simulink model "ISReferenceApplication"  (R2024b)
settings: Solver=ode5  StartTime=0.0  StopTime=20  FixedStep=1e-3  RelTol=2e-1
model workspace (MAT data in the model file):
  Downshift_Speeds = [9.5625 12.9375 16.3125 19.6875 23.0625 26.4375 29.8125 33.1875 36.5625 39.9375 43.3125 46.6875 ... (28 elements, 4x7)]
  EngRevLim = 7000
  Pedal_Positions = [0.1 0.4 0.5 0.9]
  Upshift_Speeds = [12.9375 16.3125 19.6875 33 26.4375 29.8125 33.1875 52.5 39.9375 43.3125 46.6875 77.25 ... (28 elements, 4x7)]
  VEH : object (value not decoded)
  rayDirections = [0 0 0 0 0 0 0 0 0 0 0 0 ... (363 elements, 121x3)]
  rayLengths = [20 20 20 20 20 20 20 20 20 20 20 20 ... (121 elements, 121x1)]
  rayOrigins = [0.5 0.4 0.3 0.2 0.1 0 -0.1 -0.2 -0.3 -0.4 -0.5 0.5 ... (363 elements, 121x3)]
  temp : object (value not decoded)
symbols that are objects in the model workspace (value not decoded): temp, VEH
undefined symbols (not defined in the file or in its folder): DiscIntNeverNeededParam, Sim3dSensor
libraries: simulink x28, autolibutils x14, VDriveToolbox x10, vehdynlibviscommon x4, sim3dgroundtruthsensorlib x4, slpidlib x3, autolibtranscontrolscommon x2, autolibshared x2, vehdynlibdriver x2, sharedtransform x2, vehdynlibsens x2, vehdynlibscenariocommon x2
(part 7 of 7)

== matlab function ISReferenceApplication/Visualization1/MATLAB Function ==
  data: pos input; agl input; vel input; wheel_agl input; T_ref input; track_w input; a input; b input; diameter input
function XYplot(pos,agl,vel,wheel_agl,T_ref,track_w,a,b,diameter)
persistent fig_xy ref_p
if isempty(fig_xy)
    fig_xy = figure();
    ref_p = plot(-T_ref(:,2),T_ref(:,1),'Color','red','LineWidth',1.5,'DisplayName','Ref. Path'); hold on;
end
body_yaw = agl(3);
body_x = pos(1);
body_y = pos(2);
wfl_x = body_x+a;
wfl_y = body_y-track_w/2;
wfr_x = body_x+a;
wfr_y = body_y+track_w/2;
wrl_x = body_x-b;
wrl_y = body_y-track_w/2;
wrr_x = body_x-b;
wrr_y = body_y+track_w/2;

R_whl = [cos(-wheel_agl(1)) -sin(-wheel_agl(1)) ;sin(-wheel_agl(1)) cos(-wheel_agl(1))];
R_bdy = [cos(-body_yaw) -sin(-body_yaw) ;sin(-body_yaw) cos(-body_yaw)];

wfl_rec_x = [wfl_y-0.1 wfl_y+0.1 wfl_y+0.1 wfl_y-0.1];
wfl_rec_y = [wfl_x-diameter/2 wfl_x-diameter/2 wfl_x+diameter/2 wfl_x+diameter/2];
wfr_rec_x = [wfr_y-0.1 wfr_y+0.1 wfr_y+0.1 wfr_y-0.1];
wfr_rec_y = [wfr_x-diameter/2 wfr_x-diameter/2 wfr_x+diameter/2 wfr_x+diameter/2];
wrl_rec_x = [wrl_y-0.1 wrl_y+0.1 wrl_y+0.1 wrl_y-0.1];
wrl_rec_y = [wrl_x-diameter/2 wrl_x-diameter/2 wrl_x+diameter/2 wrl_x+diameter/2];
wrr_rec_x = [wrr_y-0.1 wrr_y+0.1 wrr_y+0.1 wrr_y-0.1];
wrr_rec_y = [wrr_x-diameter/2 wrr_x-diameter/2 wrr_x+diameter/2 wrr_x+diameter/2];
bdy_rec_x = [body_y-1.731/2 body_y+1.731/2 body_y+1.731/2 body_y-1.731/2];
bdy_rec_y = [body_x-4.769/2 body_x-4.769/2 body_x+4.769/2 body_x+4.769/2];

wfl_rec = [wfl_rec_x;wfl_rec_y];
wfr_rec = [wfr_rec_x;wfr_rec_y];
wrl_rec = [wrl_rec_x;wrl_rec_y];
wrr_rec = [wrr_rec_x;wrr_rec_y];
bdy_rec = [bdy_rec_x;bdy_rec_y];

for i=1:4
    wfl_rec(:,i) = R_whl*(wfl_rec(:,i)-[wfl_y;wfl_x]) + [wfl_y;wfl_x];
    wfr_rec(:,i) = R_whl*(wfr_rec(:,i)-[wfr_y;wfr_x]) + [wfr_y;wfr_x];

    wfl_rec(:,i) = R_bdy*(wfl_rec(:,i)-[body_y;body_x]) + [body_y;body_x];
    wfr_rec(:,i) = R_bdy*(wfr_rec(:,i)-[body_y;body_x]) + [body_y;body_x];
    wrl_rec(:,i) = R_bdy*(wrl_rec(:,i)-[body_y;body_x]) + [body_y;body_x];
    wrr_rec(:,i) = R_bdy*(wrr_rec(:,i)-[body_y;body_x]) + [body_y;body_x];
    bdy_rec(:,i) = R_bdy*(bdy_rec(:,i)-[body_y;body_x]) + [body_y;body_x];
end

hold on;
bdy_sc = scatter(body_y,body_x,10,'black','filled','DisplayName','Trajectory');
txt = round(norm(vel(1:2))*3.6)+" km/h";
persistent wfl_p wfr_p wrl_p wrr_p bdy_p vel_p
if isempty(wfl_p)
bdy_p = patch(bdy_rec(1,:),bdy_rec(2,:),'black','FaceAlpha',.5); hold on;
wfl_p = patch(wfl_rec(1,:),wfl_rec(2,:),'black');
wfr_p = patch(wfr_rec(1,:),wfr_rec(2,:),'black');
wrl_p = patch(wrl_rec(1,:),wrl_rec(2,:),'black');
wrr_p = patch(wrr_rec(1,:),wrr_rec(2,:),'black');
vel_p = text(body_y-4,body_x+4,txt,'FontSize',11,'FontName','Arial');
else
    set(bdy_p,'XData',bdy_rec(1,:),'YData',bdy_rec(2,:));
    set(wfl_p,'XData',wfl_rec(1,:),'YData',wfl_rec(2,:));
    set(wfr_p,'XData',wfr_rec(1,:),'YData',wfr_rec(2,:));
    set(wrl_p,'XData',wrl_rec(1,:),'YData',wrl_rec(2,:));
    set(wrr_p,'XData',wrr_rec(1,:),'YData',wrr_rec(2,:));
    set(vel_p,'String',txt);
end

legend([ref_p,bdy_sc],{'Ref. Path','Trajectory'});

hold off;
axis('equal');
grid on;
ylim([body_x-(a+b)*2 body_x+(a+b)*2]);
xlim([body_y-(a+b)*2 body_y+(a+b)*2]);
xlabel('Y [m]'); ylabel('X [m]');

set(gca,'FontName','Arial','FontSize',11);

% coder.extrinsic('F_Video');
% F_Video();
end

== matlab function ISReferenceApplication/Driver Commands1/NLMPC using Disturbance Estimation/MATLAB Function1 ==
  data: rearAxleToCG input; initpos input; initagl input; initstate input; x input; pos output; y input; z input; roll_matlab input; pitch_matlab input; yaw_matlab input; pos input; roll input; pitch input; yaw input; roll output; pitch output; yaw output
function [pos, roll,pitch,yaw] = matlabPos2divpPos(rearAxleToCG,initpos,initagl,initstate,x,y,z,roll_matlab,pitch_matlab,yaw_matlab,pos,roll,pitch,yaw)
    R1 = eul2rotm(initagl);
    A1 = [[R1;0,0,0],[initpos(1); initpos(2); initpos(3);1]];
    divp_pos = [x-rearAxleToCG,-y,-z];
    divp_pos = A1*[divp_pos, 1]';

    pos(:,1) = divp_pos(1:3);

    yaw(1,1) = -yaw_matlab + initstate(4);
    pitch(1,1) = -pitch_matlab + initstate(5);
    roll(1,1) = roll_matlab;
end

== matlab function ISReferenceApplication/Driver Commands1/NLMPC using Disturbance Estimation/MATLAB Function9 ==
  data: NMPC input; steer_input output; last_u input
function steer_input= input_selector(NMPC, last_u)
    if ~isempty(NMPC)
        steer_input=NMPC;
    else
        steer_input = mean(last_u(1:2));
    end
end

== matlab function ISReferenceApplication/Controllers/Brake Pressure Control/Bang Bang ABS/Kappa/MATLAB Function ==
  data: Omega input; xdot input; KappaEst output
function KappaEst = fcn(Omega, xdot)

Re = 0.29;
KappaEst = 0;
WhlSpd = Omega * Re;

if xdot*WhlSpd ~= 0
    KappaEst = (WhlSpd - xdot)/max([abs(xdot) abs(WhlSpd)]);
end

== matlab function ISReferenceApplication/Driver Commands1/MATLAB Function1 ==
  data: opt_params input; rearfromCG input; T_ref input; bdy_x input; bdy_y input; phi input; x_ref output; x_dot input; y_dot input; y_ref output; yaw_ref output; vel output
function [x_ref,y_ref,yaw_ref,vel] = ReferenceGenerator(opt_params,rearfromCG,T_ref,bdy_x,bdy_y,phi,x_dot,y_dot)
    % in case of center of grabity
    x = bdy_x;
    y = -bdy_y;
    vel = norm([x_dot,y_dot]);

    % in case of Front Axle
    rear_axl = [cos(-phi) -sin(-phi); sin(-phi) cos(-phi)]*[-rearfromCG;0] + [x;y];
    rear_axl = rear_axl';
    % [k,~] = dsearchn(T_ref(:,1:2),[x,y]);
    ref = T_ref(:,1:2) - rear_axl;

    x_ref = 0:vel*opt_params.dt:vel*opt_params.dt*opt_params.N;
    y_ref = interp1(ref(:,1)',ref(:,2)',x_ref);
    yaw_ref = atan2(gradient(y_ref), gradient(x_ref));

    % current_reference = [x_ref; y_ref];

end

== matlab function ISReferenceApplication/Driver Commands1/NLMPC using Disturbance Estimation/MATLAB Function ==
  data: clock input; HitPoint input; SignalStrength input
function LidarXYZ(clock,HitPoint,SignalStrength)
    lidar_name = 'roof-lidar';
    save_dir = "pcd_"+lidar_name;

    coder.extrinsic('F_LidarXYZMap_roof');
    F_LidarXYZMap_roof(lidar_name,clock,HitPoint,SignalStrength,save_dir);
    
end

== matlab function ISReferenceApplication/Driver Commands1/NLMPC using Disturbance Estimation/MATLAB Function2 ==
  data: dc_params input; clock input; rgb input; sparse_depth input; dense_depth output
function dense_depth = depth_completion(dc_params, clock, rgb, sparse_depth)
    crop_h = dc_params.crop_h;
    crop_w = dc_params.crop_w;

    coder.extrinsic('F_depthcompletion');
    dense_depth = F_depthcompletion(clock,rgb,sparse_depth,crop_h,crop_w);
end

== matlab function ISReferenceApplication/Driver Commands1/NLMPC using Disturbance Estimation/MATLAB Function3 ==
  data: cam_params input; clock input; sparse_depth output; rgb input; lidarpoints input
function sparse_depth = pointcloud2depth(cam_params, clock, rgb, lidarpoints)

    coder.extrinsic('F_ptc2depthimg');
    sparse_depth = F_ptc2depthimg(clock, lidarpoints, rgb, cam_params);
end

== matlab function ISReferenceApplication/Driver Commands1/NLMPC using Disturbance Estimation/MATLAB Function4 ==
  data: dc_params input; clock input; img input; cropped_img output
function cropped_img = image_cropper(dc_params,clock,img)
    name = "cropped_rgb";

    coder.extrinsic('F_datacropper');
    cropped_img = F_datacropper(clock, name, img, dc_params.start_y, dc_params.start_x, dc_params.rect_height, dc_params.rect_width);
end

== matlab function ISReferenceApplication/Driver Commands1/NLMPC using Disturbance Estimation/MATLAB Function5 ==
  data: img input; dc_params input; clock input; cropped_img output
function cropped_img = image_cropper(img,dc_params,clock)
    name = "cropped_sparse_depth";

    coder.extrinsic('F_datacropper');
    cropped_img = F_datacropper(clock, name, img, dc_params.start_y, dc_params.start_x, dc_params.rect_height, dc_params.rect_width);
end

== matlab function ISReferenceApplication/Driver Commands1/NLMPC using Disturbance Estimation/MATLAB Function6 ==
  data: roll input; pitch input; yaw input; dc_params input; gradient_point output; cam_params input; depth_img input
function gradient_point = depth2gradient(roll,pitch,yaw,dc_params,cam_params,depth_img)
    % name = "";
    angle = [-yaw,-pitch,roll];

    coder.extrinsic('F_depth2gradient');
    gradient_point = F_depth2gradient(depth_img,cam_params,dc_params,angle);
end

== matlab function ISReferenceApplication/Driver Commands1/NLMPC using Disturbance Estimation/MATLAB Function7 ==
  data: opt_params input; x_ref input; y_ref input; gradient_points input; unevenness_points output
function unevenness_points = unevenness_extractor(opt_params,x_ref,y_ref,gradient_points)

    coder.extrinsic('F_points_extractor');
    unevenness_points = F_points_extractor(gradient_points,x_ref,y_ref,opt_params);
end

== matlab function ISReferenceApplication/Driver Commands1/NLMPC using Disturbance Estimation/MATLAB Function8 ==
  data: opt_params input; states input; x_ref input; y_ref input; yaw_ref input; unevenness_points input; v input; steer input; steer_cmd output
function steer_cmd = NLMPC(opt_params,states,x_ref,y_ref,yaw_ref,unevenness_points,v,steer)

    steer_fbk = mean(steer(1:2));

    coder.extrinsic('F_steering_optmizer');
    steer_cmd = F_steering_optmizer(opt_params,unevenness_points,states,x_ref,y_ref,yaw_ref,v,steer_fbk);
end

== matlab function ISReferenceApplication/Controllers/Brake Pressure Control/Five-State ABS and TCS/Wheel Accel and Slip Estimator/Kappa/MATLAB Function ==
  data: Omega input; xdot input; KappaEst output
function KappaEst = fcn(Omega, xdot)

Re = 0.29;
KappaEst = 0;
WhlSpd = Omega * Re;

if xdot*WhlSpd ~= 0
    KappaEst = (WhlSpd - xdot)/max([abs(xdot) abs(WhlSpd)]);
end

== stateflow chart ISReferenceApplication/Controllers/Brake Pressure Control/Five-State ABS and TCS/ABSCtrlForEach/For Each Subsystem/ABSForEachWheel ==
  state ABSOff
    entry:
    PbOutput = Pref;
    Flag = 0;
    during:
    PbOutput = Pref;
  state Normal
    entry:
    PbOutput = Pref;
    Flag = 0;
    during:
    PbOutput = Pref;
  state ABSOn
    state Phase1
      entry:
      PbOutput = v1;
      Flag = 1;
    state Phase5
      entry:
      PbOutput = v5;
      Flag = 5;
    state Phase2
      entry:
      PbOutput = 0;
      Flag = 2;
    state Phase4
      entry:
      PbOutput = 0;
      Flag = 4;
    state Phase3
      entry:
      PbOutput = v4;
      Flag = 3;
    (default) -> Phase1
    Phase5 -> Phase1 : [e2 < a2]
    Phase1 -> Phase2 : [e2 >= b]
    Phase4 -> Phase5 : [e2 <= a1]
    Phase2 -> Phase3 : [e2 >= A]
    Phase3 -> Phase4 : [e2 < A]
  (default) -> ABSOff
  ABSOn -> ABSOff : [abs(VehSpd) < 0.1 || Pref <= 0]
  Normal -> ABSOff [order 2] : [Pref <= 0]
  ABSOff -> Normal : [Pref > 0 && e2 < a2]
  Normal -> ABSOn [order 1] : [e1 < 0]
  data: e1 input; e2 input; PbOutput output; Flag output; b parameter; v1 parameter; v4 parameter; v5 parameter; A parameter; a2 parameter; a1 parameter; Pref input; VehSpd input
